simulink model "das"  (Simulink 6.5)
settings: Solver=ode45  StartTime=0.0  StopTime=10.0  RelTol=1e-3
libraries: cdsFilt x14, cdsRfmIO x10, cdsMuxMatrix x2, cdsEpicsOut x2, cdsOsc x1, cdsPhase x1, cdsParameters x1
settings Model: Creator=rolf  LastModifiedBy=aivanov  ExtModeAutoUpdateStatusClock=off
settings DebuggingCC: MultiTaskDSMMsg=warning  MultiTaskCondExecSysMsg=none  StrictBusMsg=None
settings RTWCC: IncludeERTFirstTime=on

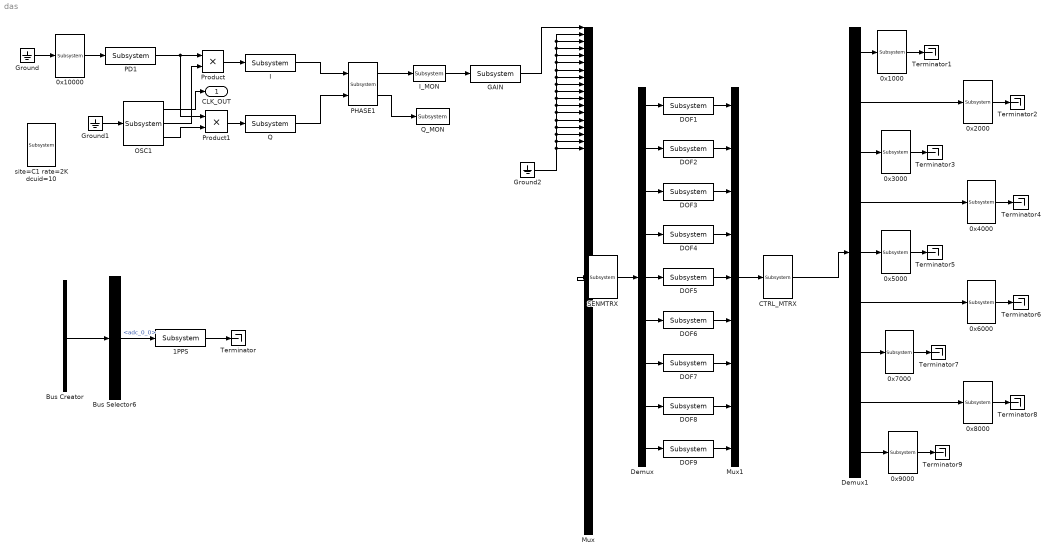
== system das ==
  0x{1000,2000,3000,4000,5000,6000,7000,8000,9000,10000} (10 alike) : cdsRfmIO/Subsystem  Tag=cdsRfmIO  Description=VMIC5565 Reflective Memory read/write  SystemSampleTime=-1
      settings: AttributesFormatString=%<Tag>
  1PPS : cdsFilt/Subsystem  Tag=cdsFilt  Description=|  SystemSampleTime=-1
      | Purpose:                                                                                                                                                                                                                                  
      | Standard CDS IIR filter module.                                                                                                                                                                                                           
      |                                                                                                                                                                                                                                           
      | Operation:                                                                                                                                                                                                                                
      | Consists of 10 second order section IIR filters, plus a ramped gain stage. In FE code, also provides pre-defined test points and excitation channel inputs. The filter coefficients are defined in the LIGO system using the 'foton' tool.
      |                                                                                                                                                                                                                                           
      | Usage:                                                                                                                                                                                                                                    
      | Name the part with the desired filter module name.
      settings: AttributesFormatString=%<Tag>
  Bus Creator : BusCreator  Inputs='adc_0_0','adc_0_1','adc_0_2','adc_0_3','adc_0_4','adc_0_5','adc_0_6','adc_0_7','adc_0_8','adc_0_9','adc_0_10','adc_0_11','adc_0_12','adc_0_13','adc_0_14','adc_0_15','adc_0_16','adc_0_17','adc_0_18','adc_0_19','adc_0_20','adc_0_21','adc_0_22','adc_0_23','adc_0_24','adc_0_25','adc_0_26','adc_0_27','adc_0_28','adc_0_29','adc_0_30','adc_0_31'
  Bus Selector6 : BusSelector  OutputSignals=adc_0_0
  CTRL_MTRX : cdsMuxMatrix/Subsystem  Tag=cdsMuxMatrix  Description=Any size matrix. Inputs and outputs must be connected using Mux and Demux parts.  SystemSampleTime=-1
      settings: AttributesFormatString=%<Tag>
  DOF1 : cdsFilt/Subsystem  Tag=cdsFilt  Description=|  SystemSampleTime=-1
      | Purpose:                                                                                                                                                                                                                                  
      | Standard CDS IIR filter module.                                                                                                                                                                                                           
      |                                                                                                                                                                                                                                           
      | Operation:                                                                                                                                                                                                                                
      | Consists of 10 second order section IIR filters, plus a ramped gain stage. In FE code, also provides pre-defined test points and excitation channel inputs. The filter coefficients are defined in the LIGO system using the 'foton' tool.
      |                                                                                                                                                                                                                                           
      | Usage:                                                                                                                                                                                                                                    
      | Name the part with the desired filter module name.
      settings: AttributesFormatString=%<Tag>
  DOF2 : cdsFilt/Subsystem  Tag=cdsFilt  Description=|  SystemSampleTime=-1
      | Purpose:                                                                                                                                                                                                                                  
      | Standard CDS IIR filter module.                                                                                                                                                                                                           
      |                                                                                                                                                                                                                                           
      | Operation:                                                                                                                                                                                                                                
      | Consists of 10 second order section IIR filters, plus a ramped gain stage. In FE code, also provides pre-defined test points and excitation channel inputs. The filter coefficients are defined in the LIGO system using the 'foton' tool.
      |                                                                                                                                                                                                                                           
      | Usage:                                                                                                                                                                                                                                    
      | Name the part with the desired filter module name.
      settings: AttributesFormatString=%<Tag>
  DOF3 : cdsFilt/Subsystem  Tag=cdsFilt  Description=|  SystemSampleTime=-1
      | Purpose:                                                                                                                                                                                                                                  
      | Standard CDS IIR filter module.                                                                                                                                                                                                           
      |                                                                                                                                                                                                                                           
      | Operation:                                                                                                                                                                                                                                
      | Consists of 10 second order section IIR filters, plus a ramped gain stage. In FE code, also provides pre-defined test points and excitation channel inputs. The filter coefficients are defined in the LIGO system using the 'foton' tool.
      |                                                                                                                                                                                                                                           
      | Usage:                                                                                                                                                                                                                                    
      | Name the part with the desired filter module name.
      settings: AttributesFormatString=%<Tag>
  DOF4 : cdsFilt/Subsystem  Tag=cdsFilt  Description=|  SystemSampleTime=-1
      | Purpose:                                                                                                                                                                                                                                  
      | Standard CDS IIR filter module.                                                                                                                                                                                                           
      |                                                                                                                                                                                                                                           
      | Operation:                                                                                                                                                                                                                                
      | Consists of 10 second order section IIR filters, plus a ramped gain stage. In FE code, also provides pre-defined test points and excitation channel inputs. The filter coefficients are defined in the LIGO system using the 'foton' tool.
      |                                                                                                                                                                                                                                           
      | Usage:                                                                                                                                                                                                                                    
      | Name the part with the desired filter module name.
      settings: AttributesFormatString=%<Tag>
  DOF5 : cdsFilt/Subsystem  Tag=cdsFilt  Description=|  SystemSampleTime=-1
      | Purpose:                                                                                                                                                                                                                                  
      | Standard CDS IIR filter module.                                                                                                                                                                                                           
      |                                                                                                                                                                                                                                           
      | Operation:                                                                                                                                                                                                                                
      | Consists of 10 second order section IIR filters, plus a ramped gain stage. In FE code, also provides pre-defined test points and excitation channel inputs. The filter coefficients are defined in the LIGO system using the 'foton' tool.
      |                                                                                                                                                                                                                                           
      | Usage:                                                                                                                                                                                                                                    
      | Name the part with the desired filter module name.
      settings: AttributesFormatString=%<Tag>
  DOF6 : cdsFilt/Subsystem  Tag=cdsFilt  Description=|  SystemSampleTime=-1
      | Purpose:                                                                                                                                                                                                                                  
      | Standard CDS IIR filter module.                                                                                                                                                                                                           
      |                                                                                                                                                                                                                                           
      | Operation:                                                                                                                                                                                                                                
      | Consists of 10 second order section IIR filters, plus a ramped gain stage. In FE code, also provides pre-defined test points and excitation channel inputs. The filter coefficients are defined in the LIGO system using the 'foton' tool.
      |                                                                                                                                                                                                                                           
      | Usage:                                                                                                                                                                                                                                    
      | Name the part with the desired filter module name.
      settings: AttributesFormatString=%<Tag>
  DOF7 : cdsFilt/Subsystem  Tag=cdsFilt  Description=|  SystemSampleTime=-1
      | Purpose:                                                                                                                                                                                                                                  
      | Standard CDS IIR filter module.                                                                                                                                                                                                           
      |                                                                                                                                                                                                                                           
      | Operation:                                                                                                                                                                                                                                
      | Consists of 10 second order section IIR filters, plus a ramped gain stage. In FE code, also provides pre-defined test points and excitation channel inputs. The filter coefficients are defined in the LIGO system using the 'foton' tool.
      |                                                                                                                                                                                                                                           
      | Usage:                                                                                                                                                                                                                                    
      | Name the part with the desired filter module name.
      settings: AttributesFormatString=%<Tag>
  DOF8 : cdsFilt/Subsystem  Tag=cdsFilt  Description=|  SystemSampleTime=-1
      | Purpose:                                                                                                                                                                                                                                  
      | Standard CDS IIR filter module.                                                                                                                                                                                                           
      |                                                                                                                                                                                                                                           
      | Operation:                                                                                                                                                                                                                                
      | Consists of 10 second order section IIR filters, plus a ramped gain stage. In FE code, also provides pre-defined test points and excitation channel inputs. The filter coefficients are defined in the LIGO system using the 'foton' tool.
      |                                                                                                                                                                                                                                           
      | Usage:                                                                                                                                                                                                                                    
      | Name the part with the desired filter module name.
      settings: AttributesFormatString=%<Tag>
  DOF9 : cdsFilt/Subsystem  Tag=cdsFilt  Description=|  SystemSampleTime=-1
      | Purpose:                                                                                                                                                                                                                                  
      | Standard CDS IIR filter module.                                                                                                                                                                                                           
      |                                                                                                                                                                                                                                           
      | Operation:                                                                                                                                                                                                                                
      | Consists of 10 second order section IIR filters, plus a ramped gain stage. In FE code, also provides pre-defined test points and excitation channel inputs. The filter coefficients are defined in the LIGO system using the 'foton' tool.
      |                                                                                                                                                                                                                                           
      | Usage:                                                                                                                                                                                                                                    
      | Name the part with the desired filter module name.
      settings: AttributesFormatString=%<Tag>
  Demux : Demux  Outputs=9
  Demux1 : Demux  Outputs=9
  GAIN : cdsFilt/Subsystem  Tag=cdsFilt  Description=|  SystemSampleTime=-1
      | Purpose:                                                                                                                                                                                                                                  
      | Standard CDS IIR filter module.                                                                                                                                                                                                           
      |                                                                                                                                                                                                                                           
      | Operation:                                                                                                                                                                                                                                
      | Consists of 10 second order section IIR filters, plus a ramped gain stage. In FE code, also provides pre-defined test points and excitation channel inputs. The filter coefficients are defined in the LIGO system using the 'foton' tool.
      |                                                                                                                                                                                                                                           
      | Usage:                                                                                                                                                                                                                                    
      | Name the part with the desired filter module name.
      settings: AttributesFormatString=%<Tag>
  Ground : Ground
  Ground1 : Ground
  Ground2 : Ground
  I : cdsFilt/Subsystem  Tag=cdsFilt  Description=|  SystemSampleTime=-1
      | Purpose:                                                                                                                                                                                                                                  
      | Standard CDS IIR filter module.                                                                                                                                                                                                           
      |                                                                                                                                                                                                                                           
      | Operation:                                                                                                                                                                                                                                
      | Consists of 10 second order section IIR filters, plus a ramped gain stage. In FE code, also provides pre-defined test points and excitation channel inputs. The filter coefficients are defined in the LIGO system using the 'foton' tool.
      |                                                                                                                                                                                                                                           
      | Usage:                                                                                                                                                                                                                                    
      | Name the part with the desired filter module name.
      settings: AttributesFormatString=%<Tag>
  I_MON : cdsEpicsOut/Subsystem  Tag=cdsEpicsOutput  Description=|  SystemSampleTime=-1
      | Purpose:                                          
      | Output a FE signal to an EPICS channel.           
      |                                                   
      | Operation:                                        
      | Takes input value and passes it to EPICS record.  
      |                                                   
      | Usage:                                            
      | Name the part with the desired EPICS rrecord name.
      settings: AttributesFormatString=%<Tag>
  Mux : Mux  Inputs=72
  Mux1 : Mux  Inputs=9
  OSC1 : cdsOsc/Subsystem  Tag=cdsOsc  Description=Oscillator  SystemSampleTime=-1
      settings: AttributesFormatString=%<Tag>
  PD1 : cdsFilt/Subsystem  Tag=cdsFilt  Description=|  SystemSampleTime=-1
      | Purpose:                                                                                                                                                                                                                                  
      | Standard CDS IIR filter module.                                                                                                                                                                                                           
      |                                                                                                                                                                                                                                           
      | Operation:                                                                                                                                                                                                                                
      | Consists of 10 second order section IIR filters, plus a ramped gain stage. In FE code, also provides pre-defined test points and excitation channel inputs. The filter coefficients are defined in the LIGO system using the 'foton' tool.
      |                                                                                                                                                                                                                                           
      | Usage:                                                                                                                                                                                                                                    
      | Name the part with the desired filter module name.
      settings: AttributesFormatString=%<Tag>
  PHASE1 : cdsPhase/Subsystem  Tag=cdsPhase  Description=Phase Rotator  SystemSampleTime=-1
      settings: AttributesFormatString=%<Tag>
  Product : Product  RndMeth=Zero
  Product1 : Product  RndMeth=Zero
  Q : cdsFilt/Subsystem  Tag=cdsFilt  Description=|  SystemSampleTime=-1
      | Purpose:                                                                                                                                                                                                                                  
      | Standard CDS IIR filter module.                                                                                                                                                                                                           
      |                                                                                                                                                                                                                                           
      | Operation:                                                                                                                                                                                                                                
      | Consists of 10 second order section IIR filters, plus a ramped gain stage. In FE code, also provides pre-defined test points and excitation channel inputs. The filter coefficients are defined in the LIGO system using the 'foton' tool.
      |                                                                                                                                                                                                                                           
      | Usage:                                                                                                                                                                                                                                    
      | Name the part with the desired filter module name.
      settings: AttributesFormatString=%<Tag>
  Q_MON : cdsEpicsOut/Subsystem  Tag=cdsEpicsOutput  Description=|  SystemSampleTime=-1
      | Purpose:                                          
      | Output a FE signal to an EPICS channel.           
      |                                                   
      | Operation:                                        
      | Takes input value and passes it to EPICS record.  
      |                                                   
      | Usage:                                            
      | Name the part with the desired EPICS rrecord name.
      settings: AttributesFormatString=%<Tag>
  SENMTRX : cdsMuxMatrix/Subsystem  Tag=cdsMuxMatrix  Description=Any size matrix. Inputs and outputs must be connected using Mux and Demux parts.  SystemSampleTime=-1
      settings: AttributesFormatString=%<Tag>
  Terminator{,1..9} (10 alike) : Terminator
  site=C1 rate=2K dcuid=10 : cdsParameters/Subsystem  Tag=cdsParameters  SystemSampleTime=-1
      settings: AttributesFormatString=%<Tag>
  CLK_OUT : Outport
  wires:
  Bus Creator/1 -> Bus Selector6/1
  Ground/1 -> 0x10000/1
  Ground1/1 -> OSC1/1
  0x10000/1 -> PD1/1
  PD1/1 -> Product/1, Product1/1
  OSC1/2 -> Product/2
  OSC1/3 -> Product1/2
  Product1/1 -> Q/1
  Product/1 -> I/1
  I/1 -> PHASE1/1
  Q/1 -> PHASE1/2
  PHASE1/1 -> I_MON/1
  PHASE1/2 -> Q_MON/1
  I_MON/1 -> GAIN/1
  GAIN/1 -> Mux/1
  OSC1/1 -> CLK_OUT/1
  Bus Selector6/1 -> 1PPS/1  "<adc_0_0>"
  1PPS/1 -> Terminator/1
  Mux/1 -> SENMTRX/1
  SENMTRX/1 -> Demux/1
  Demux/1 -> DOF1/1
  Demux/2 -> DOF2/1
  Demux/3 -> DOF3/1
  Demux/4 -> DOF4/1
  Demux/5 -> DOF5/1
  Demux/6 -> DOF6/1
  Demux/7 -> DOF7/1
  Demux/8 -> DOF8/1
  Demux/9 -> DOF9/1
  Mux1/1 -> CTRL_MTRX/1
  CTRL_MTRX/1 -> Demux1/1
  DOF1/1 -> Mux1/1
  DOF2/1 -> Mux1/2
  DOF3/1 -> Mux1/3
  DOF4/1 -> Mux1/4
  DOF5/1 -> Mux1/5
  DOF6/1 -> Mux1/6
  DOF7/1 -> Mux1/7
  DOF8/1 -> Mux1/8
  DOF9/1 -> Mux1/9
  Demux1/1 -> 0x1000/1
  0x1000/1 -> Terminator1/1
  0x2000/1 -> Terminator2/1
  Demux1/2 -> 0x2000/1
  0x3000/1 -> Terminator3/1
  Demux1/3 -> 0x3000/1
  0x4000/1 -> Terminator4/1
  Demux1/4 -> 0x4000/1
  0x5000/1 -> Terminator5/1
  0x6000/1 -> Terminator6/1
  0x7000/1 -> Terminator7/1
  0x8000/1 -> Terminator8/1
  0x9000/1 -> Terminator9/1
  Demux1/5 -> 0x5000/1
  Demux1/6 -> 0x6000/1
  Demux1/7 -> 0x7000/1
  Demux1/8 -> 0x8000/1
  Demux1/9 -> 0x9000/1
  Ground2/1 -> Mux/9, Mux/4, Mux/2, Mux/3, Mux/5, Mux/6, Mux/7, Mux/8, Mux/10, Mux/11, Mux/12, Mux/13, Mux/14, Mux/15, Mux/16, Mux/17, Mux/18
